simulink model "SimpleInputOutputSchematic"  (R2022a)
settings: Solver=VariableStepAuto  StartTime=0.0  StopTime=10.0  RelTol=1e-3
settings Model: Creator=feyzi  LastModifiedBy=feyzi

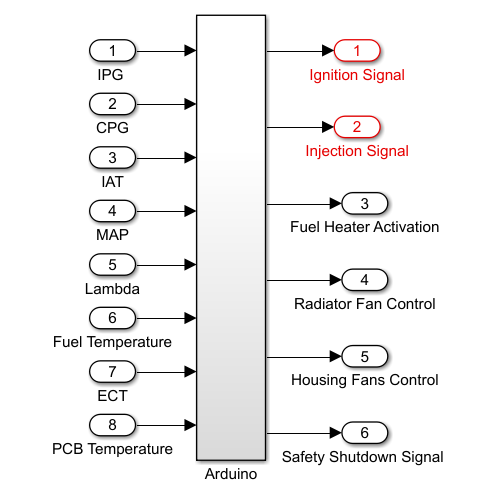
[thumbnail: Simulink's stored preview of the top-level diagram]
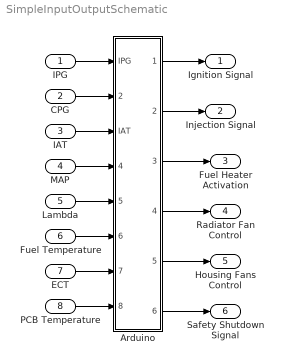
== system SimpleInputOutputSchematic ==
  "IPG " : Inport
  CPG : Inport  Port=2
  IAT : Inport  Port=3
  MAP : Inport  Port=4
  Lambda : Inport  Port=5
  Fuel Temperature : Inport  Port=6
  ECT : Inport  Port=7
  PCB Temperature : Inport  Port=8
  Arduino : Subsystem
  Ignition Signal : Outport
  Injection Signal : Outport  Port=2
  Fuel Heater Activation : Outport  Port=3
  Radiator Fan Control : Outport  Port=4
  Housing Fans Control : Outport  Port=5
  "Safety Shutdown Signal " : Outport  Port=6
  wires:
  "IPG "/1 -> Arduino/1("IPG ")
  CPG/1 -> Arduino/2(CPG)
  IAT/1 -> Arduino/3(IAT)
  MAP/1 -> Arduino/4(MAP)
  Lambda/1 -> Arduino/5(Lambda)
  Fuel Temperature/1 -> Arduino/6(Fuel Temperature)
  ECT/1 -> Arduino/7(ECT)
  PCB Temperature/1 -> Arduino/8(PCB Temperature)
  Arduino/1(Ignition Signal) -> Ignition Signal/1
  Arduino/2(Injection Signal) -> Injection Signal/1
  Arduino/3(Fuel Heater) -> Fuel Heater Activation/1
  Arduino/4(Radiator fans) -> Radiator Fan Control/1
  Arduino/5(Housing Fans) -> Housing Fans Control/1
  Arduino/6("Safety Shutdown Signal ") -> "Safety Shutdown Signal "/1

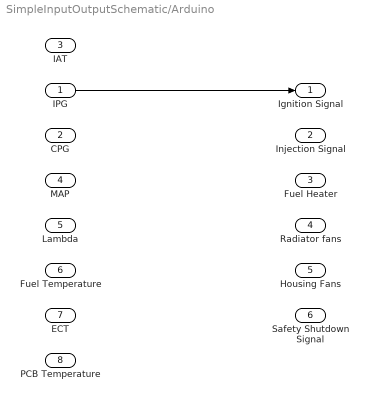
== system SimpleInputOutputSchematic/Arduino ==
  "IPG " : Inport
  CPG : Inport  Port=2
  IAT : Inport  Port=3
  MAP : Inport  Port=4
  Lambda : Inport  Port=5
  Fuel Temperature : Inport  Port=6
  ECT : Inport  Port=7
  PCB Temperature : Inport  Port=8
  Ignition Signal : Outport
  Injection Signal : Outport  Port=2
  Fuel Heater : Outport  Port=3
  Radiator fans : Outport  Port=4
  Housing Fans : Outport  Port=5
  "Safety Shutdown Signal " : Outport  Port=6
  wires:
  "IPG "/1 -> Ignition Signal/1
